simulink model "LAB_Enco002"  (R2024b)
settings: Solver=FixedStepAuto  StartTime=0.0  StopTime=inf  FixedStep=0.01  RelTol=1e-3  EnableMultiTasking=on
libraries: stm32g4xxblockslib x3, stm32f4xxblockslib x2
settings Model: STM32="{\"DigitalPortRead\":[{\"ID\":\"untitled:5\"},{\"ID\":\"untitled:6\"},{\"ID\":\"LAB_Enco002:5\"},{\"ID\":\"LAB_Enco002:36\"}],\"EncoderBlockForG4\":[{\"ID\":\"untitled:21\"},{\"ID\":\"untitled:22\"},{\"ID\":\"untitled:23\"},{\"ID\":\"LAB_Enco002:21\"},{\"ID\":\"LAB_Enco002:22\"},{\"ID\":\"LAB_Enco002:23\"}]}"  Creator=rachc  LastModifiedBy=rachc
settings OptimizationCC: DefaultParameterBehavior=Inlined  EnhancedBackFolding=on  PassReuseOutputArgsAs=Individual arguments  ZeroExternalMemoryAtStartup=off  ZeroInternalMemoryAtStartup=off  MaxStackSize=512  OptimizeBlockOrder=speed  DifferentSizesBufferReuse=on  OptimizationCustomize=off  EfficientTunableParamExpr=on
settings DebuggingCC: ParameterTunabilityLossMsg=error
settings HardwareCC: ProdBitPerPointer=32  ProdBitPerSizeT=32  ProdBitPerPtrDiffT=32  ProdLargestAtomicInteger=Long  ProdLargestAtomicFloat=Double  ProdWordSize=32  ProdHWDeviceType=ARM Compatible->ARM Cortex-M
settings SFSimCC: MATLABDynamicMemAlloc=off
settings RTWCC: Description=Embedded Coder  SystemTargetFile=ert.tlc  HardwareBoard=STM32G4xx Based  TemplateMakefile=ert_default_tmf  Toolchain=GNU Tools for ARM Embedded Processors
settings CodeAppCC: ForceParamTrailComments=on  IgnoreCustomStorageClasses=off  OperatorAnnotations=on  SimulinkDataObjDesc=on  SFDataObjDesc=on  InsertBlockDesc=on
settings ERTTargetCC: TargetLangStandard=C99 (ISO)  CodeReplacementLibrary=ARM Cortex-M  ExtModeTransport=3  ExtModeStaticAlloc=on  ExtModeStaticAllocSize=2048  ExtModeMexFile=ext_xcp  ExtModeIntrfLevel=Level2 - Open

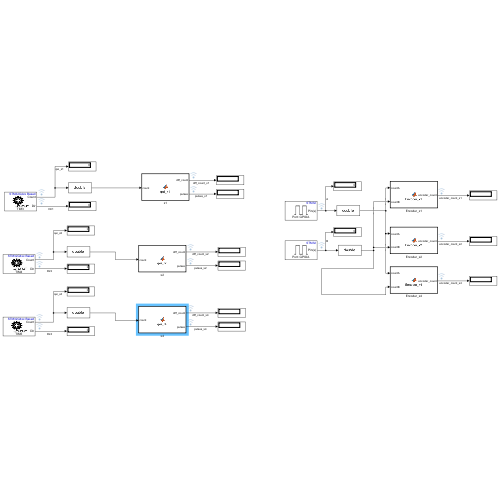
[thumbnail: Simulink's stored preview of the top-level diagram]
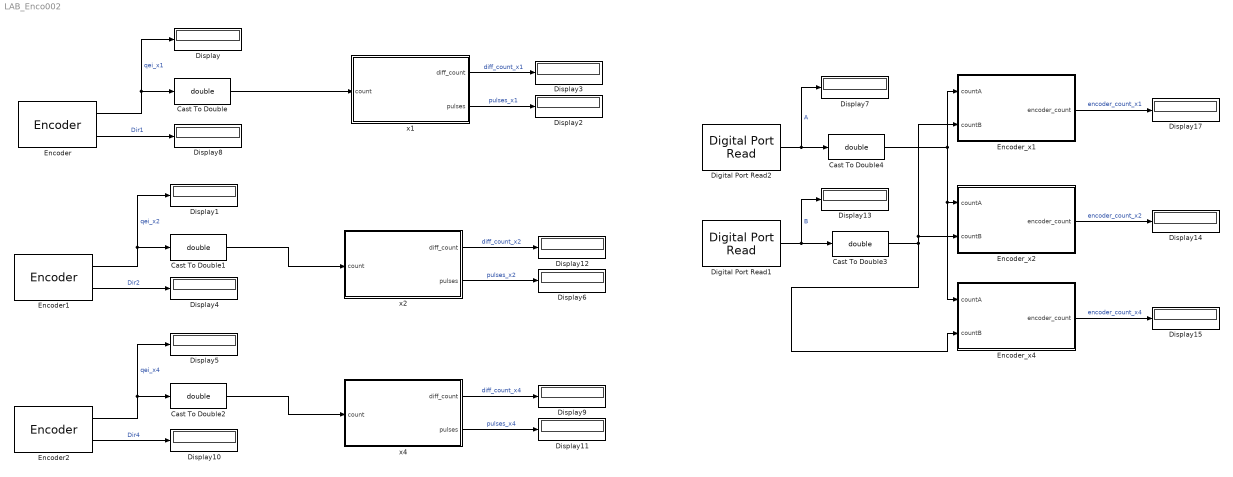
== system LAB_Enco002 ==
  Cast To Double{,1..4} (5 alike) : DataTypeConversion  OutDataTypeStr=double  SaturateOnIntegerOverflow=off  RndMeth=Floor
  Digital Port Read1 : stm32f4xxblockslib/Digital Port Read  PortName=GPIOA  PinNumber=7  ReadOperation=on  IOAsArray=on  SampleTime=-1  EnableSimPort=off  hoistedMaskSrc=ECSoC/ECSimCodegen/Digital Port Read
      settings: LibrarySourceBlock=stm32g4xxblockslib/Digital Port Read
  Digital Port Read2 : stm32f4xxblockslib/Digital Port Read  PortName=GPIOA  PinNumber=6  ReadOperation=on  IOAsArray=on  SampleTime=-1  EnableSimPort=off  hoistedMaskSrc=ECSoC/ECSimCodegen/Digital Port Read
      settings: LibrarySourceBlock=stm32g4xxblockslib/Digital Port Read
  Display{,1..15,17} (17 alike) : Display
  Encoder : stm32g4xxblockslib/Encoder  TimerModule=TIM3  EnableResetInput=off  OutputCountAfterFirstIndex=off  OutputValidIndex=off  OutputDirection=on  OutputStatus=off  SampleTime=-1
  Encoder1 : stm32g4xxblockslib/Encoder  TimerModule=TIM4  EnableResetInput=off  OutputCountAfterFirstIndex=off  OutputValidIndex=off  OutputDirection=on  OutputStatus=off  SampleTime=-1
  Encoder2 : stm32g4xxblockslib/Encoder  TimerModule=TIM5  EnableResetInput=off  OutputCountAfterFirstIndex=off  OutputValidIndex=off  OutputDirection=on  OutputStatus=off  SampleTime=-1
  Encoder_x1 : MATLAB Function  TreatAsAtomicUnit=on
  Encoder_x2 : MATLAB Function  TreatAsAtomicUnit=on
  Encoder_x4 : MATLAB Function  TreatAsAtomicUnit=on
  x1 : MATLAB Function  TreatAsAtomicUnit=on
  x2 : MATLAB Function  TreatAsAtomicUnit=on
  x4 : MATLAB Function  TreatAsAtomicUnit=on
  wires:
  Cast To Double1/1 -> x2/1(count)
  x1/2(pulses) -> Display2/1  "pulses_x1"
  x2/2(pulses) -> Display6/1  "pulses_x2"
  Encoder2/2 -> Display10/1  "Dir4"
  Digital Port Read1/1 -> Cast To Double3/1, Display13/1  "B"
  Encoder/1 -> Cast To Double/1, Display/1  "qei_x1"
  Encoder1/1 -> Cast To Double1/1, Display1/1  "qei_x2"
  Encoder2/1 -> Cast To Double2/1, Display5/1  "qei_x4"
  x4/1(diff_count) -> Display9/1  "diff_count_x4"
  x4/2(pulses) -> Display11/1  "pulses_x4"
  Digital Port Read2/1 -> Display7/1, Cast To Double4/1  "A"
  x2/1(diff_count) -> Display12/1  "diff_count_x2"
  x1/1(diff_count) -> Display3/1  "diff_count_x1"
  Encoder/2 -> Display8/1  "Dir1"
  Cast To Double/1 -> x1/1(count)
  Cast To Double2/1 -> x4/1(count)
  Encoder1/2 -> Display4/1  "Dir2"
  Encoder_x1/1(encoder_count) -> Display17/1  "encoder_count_x1"
  Cast To Double3/1 -> Encoder_x4/2(countB), Encoder_x2/2(countB), Encoder_x1/2(countB)
  Cast To Double4/1 -> Encoder_x4/1(countA), Encoder_x2/1(countA), Encoder_x1/1(countA)
  Encoder_x2/1(encoder_count) -> Display14/1  "encoder_count_x2"
  Encoder_x4/1(encoder_count) -> Display15/1  "encoder_count_x4"

== matlab function LAB_Enco002/x1 ==
  data: count input; diff_count output; pulses output
function [diff_count,pulses]  = qei_x1(count)
persistent prev_count 
persistent prev_pulses
enc = 65520;

    if isempty(prev_count)
        prev_count = 0;
    end
    if isempty(prev_pulses)
        prev_pulses = 0;
    end

    diff_count = count- prev_count;
    if diff_count > enc / 2
        diff_count = diff_count - enc;
    elseif diff_count < -enc / 2
        diff_count = diff_count + enc;
    end
    
    prev_pulses = prev_pulses + diff_count;
    prev_count = count;
    pulses = prev_pulses
    
end

== matlab function LAB_Enco002/x4 ==
  data: count input; diff_count output; pulses output
function [diff_count,pulses]  = qei_x4(count)
persistent prev_count 
persistent prev_pulses
enc = 65520;

    if isempty(prev_count)
        prev_count = 0;
    end
    if isempty(prev_pulses)
        prev_pulses = 0;
    end

    diff_count = count- prev_count;
    if diff_count > enc / 2
        diff_count = diff_count - enc;
    elseif diff_count < -enc / 2
        diff_count = diff_count + enc;
    end
    
    prev_pulses = prev_pulses + diff_count;
    prev_count = count;
    pulses = prev_pulses
    
end

== matlab function LAB_Enco002/x2 ==
  data: count input; diff_count output; pulses output
function [diff_count,pulses]  = qei_x2(count)
persistent prev_count 
persistent prev_pulses
enc = 65520;

    if isempty(prev_count)
        prev_count = 0;
    end
    if isempty(prev_pulses)
        prev_pulses = 0;
    end

    diff_count = count- prev_count;
    if diff_count > enc / 2
        diff_count = diff_count - enc;
    elseif diff_count < -enc / 2
        diff_count = diff_count + enc;
    end
    
    prev_pulses = prev_pulses + diff_count;
    prev_count = count;
    pulses = prev_pulses
    
end

== matlab function LAB_Enco002/Encoder_x1 ==
  data: countA input; encoder_count output; countB input
function encoder_count = Encoder_x1(countA, countB)
persistent prev_countA prev_pulses
if isempty(prev_countA)prev_countA = countA;end
if isempty(prev_pulses)prev_pulses = 0;end    

diff_countA = countA - prev_countA;
if diff_countA == -1
     if countB == 1
          prev_pulses = prev_pulses + 1; 
     else
          prev_pulses = prev_pulses - 1;
     end
else
   prev_pulses = prev_pulses;
 
end

encoder_count = prev_pulses;
prev_countA = countA;

end

== matlab function LAB_Enco002/Encoder_x2 ==
  data: countA input; encoder_count output; countB input
function encoder_count = Encoder_x2(countA, countB)
    persistent prev_countA prev_pulses
    if isempty(prev_countA), prev_countA = countA; end
    if isempty(prev_pulses), prev_pulses = 0; end

    if countA ~= prev_countA
        if countA ~= countB
            prev_pulses = prev_pulses + 1;
        else
            prev_pulses = prev_pulses - 1;
        end
    end

    encoder_count = prev_pulses;
    prev_countA = countA;
end

== matlab function LAB_Enco002/Encoder_x4 ==
  data: countA input; encoder_count output; countB input
function encoder_count = Encoder_x4(countA, countB)
    persistent prev_countA prev_countB prev_pulses
    if isempty(prev_countA), prev_countA = countA; end
    if isempty(prev_countB), prev_countB = countB; end
    if isempty(prev_pulses), prev_pulses = 0; end

    
    if countA ~= prev_countA
         if countA ~= countB
              prev_pulses = prev_pulses + 1;
         else
              prev_pulses = prev_pulses -1;
         end
    end
    if countB ~= prev_countB
         if countB == countA
              prev_pulses = prev_pulses +1;
         else
              prev_pulses = prev_pulses -1;
         end
    end

    encoder_count = prev_pulses;
    prev_countA = countA;
    prev_countB = countB;
end
